simulink model "vocoder"  (R2020a)
settings: Solver=FixedStepDiscrete  StartTime=0.0  StopTime=inf  RelTol=1e-3
libraries: dspvision x3, audiosources x2, dspstat3 x2, dspsnks4 x1
settings Model: Creator=unity  LastModifiedBy=unity
settings SolverCC: AutoInsertRateTranBlk=on
settings DataIOCC: LimitDataPoints=on  SaveOutput=off  SignalLogging=off  SaveTime=off
settings OptimizationCC: LifeSpan=inf
settings DebuggingCC: AlgebraicLoopMsg=error  SingleTaskRateTransMsg=error  AllowSymbolicDim=off  SFUnexpectedBacktrackingDiag=warning  SFNoUnconditionalDefaultTransitionDiag=warning  SFExecutionAtInitializationDiag=none  UnderSpecifiedDimensionMsg=warning  ArithmeticOperatorsInVariantConditions=warning
settings SFSimCC: SimUseLocalCustomCode=off  CustomCodeUndefinedFunction=UseInterfaceOnly
settings RTWCC: RTWUseLocalCustomCode=off
settings CodeAppCC: StateflowObjectComments=on
settings GRTTargetCC: TargetLangStandard=C89/C90 (ANSI)
settings ConfigComp: CovMetricSettings=dw  CovHtmlReporting=on  CovSaveCumulativeToWorkspaceVar=on  CovSaveSingleToWorkspaceVar=on  CovExternalEMLEnable=off  CovSFcnEnable=off

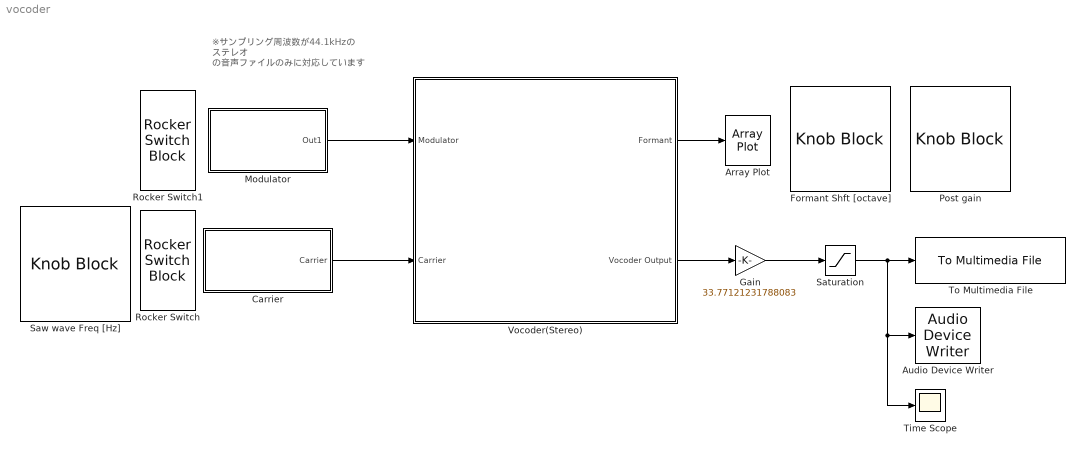
== system vocoder ==
  note: ※サンプリング周波数が44.1kHzの ステレオ の音声ファイルのみに対応しています
  Array Plot : ArrayPlot
  Audio Device Writer : dspsnks4/Audio Device Writer  Driver=DirectSound  Device=Default  InheritSampleRate=on  SampleRate=44100  BitDepth=16-bit integer  BufferSize=4096  NumBuffers=10  DefaultOutputChannelMapping=on  OutputChannelMapping=1:2  OutputNumUnderrunSamples=off  DriverIdx=1  DeviceWarnFlag=''
  Carrier : Subsystem
  Formant Shft [octave] : KnobBlock  LabelPosition=Hide  ScaleMin=-3  ScaleMax=3
  Gain : Gain  Gain=33.77121231788083
  Modulator : Subsystem
  Post gain : KnobBlock  LabelPosition=Hide  ScaleMin=1  ScaleType=Log
  Rocker Switch : RockerSwitchBlock  LabelPosition=Hide
      settings: Values={{'Audio File', 'Saw'}, [1 0]}
  Rocker Switch1 : RockerSwitchBlock  LabelPosition=Hide
      settings: Values={{'Audio File', 'Mic.'}, [1 0]}
  Saturation : Saturate  UpperLimit=1  LowerLimit=-1
  Saw wave Freq [Hz] : KnobBlock  LabelPosition=Hide  ScaleMin=10  ScaleMax=1000  ScaleType=Log
  Time Scope : Scope
  To Multimedia File : dspvision/To Multimedia File  outputFilename=output.wav  streamSelection=Audio only  videoCompressor=None (uncompressed)  audioCompressor=None (uncompressed)  imagePorts=Separate color signals  fileType=WAV  audioDatatype=24-bit integer  fourcc=RGB  videoQuality=75  mj2000CompFactor=10
  Vocoder(Stereo) : Subsystem
  wires:
  Vocoder(Stereo)/1(Formant) -> Array Plot/1
  Vocoder(Stereo)/2(Vocoder Output) -> Gain/1
  Gain/1 -> Saturation/1
  Carrier/1(Carrier) -> Vocoder(Stereo)/2(Carrier)
  Saturation/1 -> To Multimedia File/1, Time Scope/1, Audio Device Writer/1
  Modulator/1(Out1) -> Vocoder(Stereo)/1(Modulator)

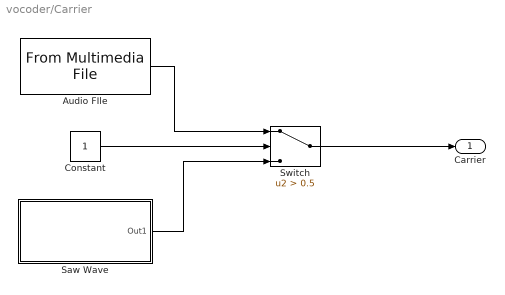
== system vocoder/Carrier ==
  Audio FIle : dspvision/From Multimedia File  inputFilename=audio_resource\carrier.wav  readRange=[1 Inf]  loop=on  numPlays=inf  outputStreams=オーディオのみ  videoDataType=single  audioDataType=double  inheritSampleTime=on  userDefinedSampleTime=1/30  noAudioOutput=off  isIntensityVideo=off  fourcc=RGB  colorVideoFormat=Separate color signals  outputEOF=off  dataOrg=Column-major  audioFrameSize=1024  computeAudioFrameSize=off  outSamplingMode=Sample based
  Constant : Constant
  Saw Wave : Subsystem
  Switch : Switch  Criteria=u2 > Threshold  Threshold=0.5
  Carrier : Outport
  wires:
  Switch/1 -> Carrier/1
  Constant/1 -> Switch/2
  Saw Wave/1(Out1) -> Switch/3
  Audio FIle/1 -> Switch/1

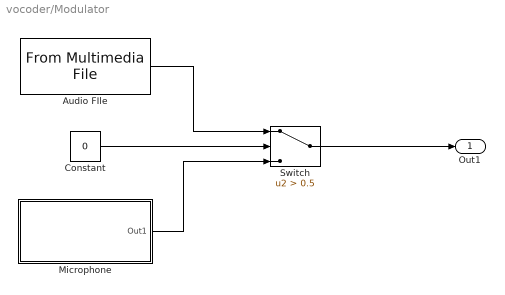
== system vocoder/Modulator ==
  Audio FIle : dspvision/From Multimedia File  inputFilename=audio_resource\modulator.wav  readRange=[1 Inf]  loop=on  numPlays=inf  outputStreams=オーディオのみ  videoDataType=single  audioDataType=double  inheritSampleTime=on  userDefinedSampleTime=1/30  noAudioOutput=off  isIntensityVideo=off  fourcc=RGB  colorVideoFormat=Separate color signals  outputEOF=off  dataOrg=Column-major  audioFrameSize=1024  computeAudioFrameSize=off  outSamplingMode=Sample based
  Constant : Constant  Value=0
  Microphone : Subsystem
  Switch : Switch  Criteria=u2 > Threshold  Threshold=0.5
  Out1 : Outport
  wires:
  Microphone/1(Out1) -> Switch/3
  Constant/1 -> Switch/2
  Switch/1 -> Out1/1
  Audio FIle/1 -> Switch/1

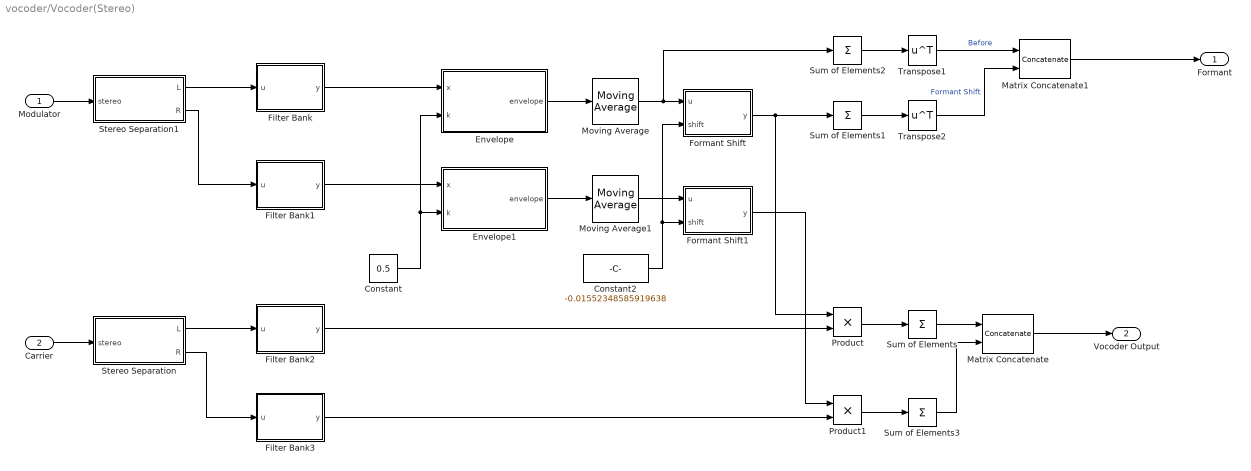
== system vocoder/Vocoder(Stereo) ==
  Modulator : Inport
  Carrier : Inport  Port=2
  Constant : Constant  Value=0.5
  Constant2 : Constant  Value=-0.01552348585919638
  Envelope : MATLAB Function  TreatAsAtomicUnit=on
  Envelope1 : MATLAB Function  TreatAsAtomicUnit=on
  Filter Bank : MATLAB Function  TreatAsAtomicUnit=on
  Filter Bank1 : MATLAB Function  TreatAsAtomicUnit=on
  Filter Bank2 : MATLAB Function  TreatAsAtomicUnit=on
  Filter Bank3 : MATLAB Function  TreatAsAtomicUnit=on
  Formant Shift : MATLAB Function  TreatAsAtomicUnit=on
  Formant Shift1 : MATLAB Function  TreatAsAtomicUnit=on
  Matrix Concatenate : Concatenate  Mode=Multidimensional array  ConcatenateDimension=2
  Matrix Concatenate1 : Concatenate  Mode=Multidimensional array  ConcatenateDimension=2
  Moving Average : dspstat3/Moving Average  Method=Sliding window  ForgettingFactorPort=off  SpecifyWindowLength=on  WindowLength=500  ForgettingFactor=0.9  SimulateUsing=Code generation
  Moving Average1 : dspstat3/Moving Average  Method=Sliding window  ForgettingFactorPort=off  SpecifyWindowLength=on  WindowLength=500  ForgettingFactor=0.9  SimulateUsing=Code generation
  Product : Product
  Product1 : Product
  Stereo Separation : MATLAB Function  TreatAsAtomicUnit=on
  Stereo Separation1 : MATLAB Function  TreatAsAtomicUnit=on
  Sum of Elements : Sum  Inputs=+  CollapseMode=Specified dimension  CollapseDim=2
  Sum of Elements1 : Sum  Inputs=+  CollapseMode=Specified dimension
  Sum of Elements2 : Sum  Inputs=+  CollapseMode=Specified dimension
  Sum of Elements3 : Sum  Inputs=+  CollapseMode=Specified dimension  CollapseDim=2
  Transpose1 : Math  Operator=transpose  SaturateOnIntegerOverflow=on
  Transpose2 : Math  Operator=transpose  SaturateOnIntegerOverflow=on
  Formant : Outport
  Vocoder Output : Outport  Port=2
  wires:
  Envelope1/1(envelope) -> Moving Average1/1
  Product/1 -> Sum of Elements/1
  Product1/1 -> Sum of Elements3/1
  Constant/1 -> Envelope1/2(k), Envelope/2(k)
  Moving Average/1 -> Sum of Elements2/1, Formant Shift/1(u)
  Envelope/1(envelope) -> Moving Average/1
  Sum of Elements1/1 -> Transpose2/1
  Filter Bank2/1(y) -> Product/2
  Filter Bank1/1(y) -> Envelope1/1(x)
  Constant2/1 -> Formant Shift/2(shift), Formant Shift1/2(shift)
  Formant Shift/1(y) -> Sum of Elements1/1, Product/1
  Matrix Concatenate1/1 -> Formant/1
  Sum of Elements2/1 -> Transpose1/1
  Stereo Separation/2(R) -> Filter Bank3/1(u)
  Formant Shift1/1(y) -> Product1/1
  Filter Bank/1(y) -> Envelope/1(x)
  Filter Bank3/1(y) -> Product1/2
  Transpose1/1 -> Matrix Concatenate1/1  "Before"
  Stereo Separation/1(L) -> Filter Bank2/1(u)
  Sum of Elements/1 -> Matrix Concatenate/1
  Sum of Elements3/1 -> Matrix Concatenate/2
  Stereo Separation1/1(L) -> Filter Bank/1(u)
  Moving Average1/1 -> Formant Shift1/1(u)
  Modulator/1 -> Stereo Separation1/1(stereo)
  Stereo Separation1/2(R) -> Filter Bank1/1(u)
  Transpose2/1 -> Matrix Concatenate1/2  "Formant Shift"
  Carrier/1 -> Stereo Separation/1(stereo)
  Matrix Concatenate/1 -> Vocoder Output/1

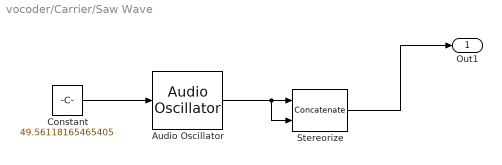
== system vocoder/Carrier/Saw Wave ==
  Audio Oscillator : audiosources/Audio Oscillator  FrequencyPort=on  Frequency=150  AmplitudePort=off  Amplitude=0.8  DCOffsetPort=off  PhaseOffset=0  DCOffset=0  WidthPort=off  Width=1  DutyCyclePort=off  DutyCycle=0.5  SampsPerFrame=1024  Fs=44100  OutputDataType=double  SimulateUsing=Code generation
      settings: SourceProductBaseCode=AU  SignalType=sawtooth
  Constant : Constant  Value=49.56118165465405
  Stereorize : Concatenate  Mode=Multidimensional array  ConcatenateDimension=2
  Out1 : Outport
  wires:
  Audio Oscillator/1 -> Stereorize/2, Stereorize/1
  Stereorize/1 -> Out1/1
  Constant/1 -> Audio Oscillator/1

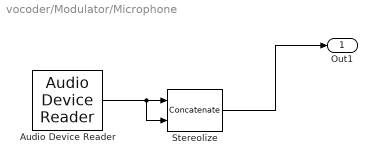
== system vocoder/Modulator/Microphone ==
  Audio Device Reader : audiosources/Audio Device Reader  Driver=DirectSound  Device=Default  SampleRate=44100  NumChannels=1  SamplesPerFrame=1024  BitDepth=16-bit integer  NumBuffers=10  DefaultInputChannelMapping=on  InputChannelMapping=1:2  OutputNumOverrunSamples=off  OutputDataType=double  DriverIdx=1  DeviceWarnFlag=''
      settings: SourceProductBaseCode=AU
  Stereolize : Concatenate  Mode=Multidimensional array  ConcatenateDimension=2
  Out1 : Outport
  wires:
  Audio Device Reader/1 -> Stereolize/2, Stereolize/1
  Stereolize/1 -> Out1/1

== matlab function vocoder/Vocoder(Stereo)/Filter Bank ==
  data: u input; y output
function y = fcn(u)
    
    persistent ofb
    if isempty(ofb)
        ofb = octaveFilterBank('1/6 octave',"FilterOrder",4);
    end

    %フィルタバンクの適用
    y = ofb(u);

== matlab function vocoder/Vocoder(Stereo)/Filter Bank1 ==
  data: u input; y output
function y = fcn(u)
    
    persistent ofb
    if isempty(ofb)
        ofb = octaveFilterBank('1/6 octave',"FilterOrder",4);
    end

    %フィルタバンクの適用
    y = ofb(u);

== matlab function vocoder/Vocoder(Stereo)/Formant Shift ==
  data: u input; y output; shift input
function y  = fcn(u,shift)
    %フレームサイズと帯域の分割数を取得
    [frame_size,n_bands]=size(u);
    
    %エンヴェロープの左右に余白を取る（エンヴェロープの配列と同じ大きさのゼロ行列を結合）
    v = cat(2,cat(2,zeros(frame_size,n_bands),u),zeros(frame_size,n_bands));
    
    %フォルマントシフト後の配列の始めの要素が，フォルマントシフト前のどの要素だったのかを取得
    %余白を取った分，n_bandsだけ平行移動している
    %オクターブフィルタが1/6 octaveなので，6を掛けて単位をオクターブにそろえる
    %マトラボでは始めの要素は１なので，１を足す
    p = n_bands-shift*6+1;
    
    %整数部分の計算
    p_int = floor(p);
    
    %小数部分の計算
    p_dec = p - p_int;
    
    %二つの配列のブレンド
    y = v(:,(p_int):(p_int+n_bands-1))*(1-p_dec)+v(:,(p_int+1):(p_int+n_bands))*p_dec;

== matlab function vocoder/Vocoder(Stereo)/Filter Bank2 ==
  data: u input; y output
function y = fcn(u)
    
    persistent ofb
    if isempty(ofb)
        ofb = octaveFilterBank('1/6 octave',"FilterOrder",4);
    end

    %フィルタバンクの適用
    y = ofb(u);

== matlab function vocoder/Vocoder(Stereo)/Stereo Separation ==
  data: stereo input; L output; R output
function [L,R] = fcn(stereo)
    L = stereo(:,1);
    R = stereo(:,2);

== matlab function vocoder/Vocoder(Stereo)/Stereo Separation1 ==
  data: stereo input; L output; R output
function [L,R] = fcn(stereo)
    L = stereo(:,1);
    R = stereo(:,2);

== matlab function vocoder/Vocoder(Stereo)/Envelope1 ==
  data: x input; envelope output; k input
function envelope = fcn(x,k)
    %入力の配列のサイズから帯域数n_bandsとframe_sizeを求める
    [n_bands,frame_size]=size(x);

    %現在のエンヴェロープの値を保存する永続な配列yの作成
    persistent y
    if isempty(y)
        y = zeros(n_bands);
    end

    %入力の絶対値を取る
    x = abs(x);

    %エンヴェロープの配列の初期化
    envelope = zeros(n_bands,frame_size);

    %全体域にわたる繰り返し
    for band = 1:n_bands
        %全サンプルにわたる繰り返し
        for i = 1:frame_size
            %yの値の更新
            if y(band) <= x(band,i)
                y(band) = x(band,i);
            else
                y(band) = y(band)*k;
            end
            envelope(band,i) = y(band);
        end
    end
end

== matlab function vocoder/Vocoder(Stereo)/Formant Shift1 ==
  data: u input; y output; shift input
function y  = fcn(u,shift)
    %フレームサイズと帯域の分割数を取得
    [frame_size,n_bands]=size(u);
    
    %エンヴェロープの左右に余白を取る（エンヴェロープの配列と同じ大きさのゼロ行列を結合）
    v = cat(2,cat(2,zeros(frame_size,n_bands),u),zeros(frame_size,n_bands));
    
    %フォルマントシフト後の配列の始めの要素が，フォルマントシフト前のどの要素だったのかを取得
    %余白を取った分，n_bandsだけ平行移動している
    %オクターブフィルタが1/6 octaveなので，6を掛けて単位をオクターブにそろえる
    %マトラボでは始めの要素は１なので，１を足す
    p = n_bands-shift*6+1;
    
    %整数部分の計算
    p_int = floor(p);
    
    %小数部分の計算
    p_dec = p - p_int;
    
    %二つの配列のブレンド
    y = v(:,(p_int):(p_int+n_bands-1))*(1-p_dec)+v(:,(p_int+1):(p_int+n_bands))*p_dec;

== matlab function vocoder/Vocoder(Stereo)/Filter Bank3 ==
  data: u input; y output
function y = fcn(u)
    
    persistent ofb
    if isempty(ofb)
        ofb = octaveFilterBank('1/6 octave',"FilterOrder",4);
    end

    %フィルタバンクの適用
    y = ofb(u);

== matlab function vocoder/Vocoder(Stereo)/Envelope ==
  data: x input; envelope output; k input
function envelope = fcn(x,k)
    %入力の配列のサイズから帯域数n_bandsとframe_sizeを求める
    [n_bands,frame_size]=size(x);

    %現在のエンヴェロープの値を保存する永続な配列yの作成
    persistent y
    if isempty(y)
        y = zeros(n_bands);
    end

    %入力の絶対値を取る
    x = abs(x);

    %エンヴェロープの配列の初期化
    envelope = zeros(n_bands,frame_size);

    %全体域にわたる繰り返し
    for band = 1:n_bands
        %全サンプルにわたる繰り返し
        for i = 1:frame_size
            %yの値の更新
            if y(band) <= x(band,i)
                y(band) = x(band,i);
            else
                y(band) = y(band)*k;
            end
            envelope(band,i) = y(band);
        end
    end
end
